simulink model "spwm_3_class3"  (R2024b)
settings: Solver=VariableStepAuto  StartTime=0.0  StopTime=1/50  RelTol=1e-3
libraries: spsTriangleGeneratorLib x1
settings Model: Creator=vasudha  LastModifiedBy=vasudha

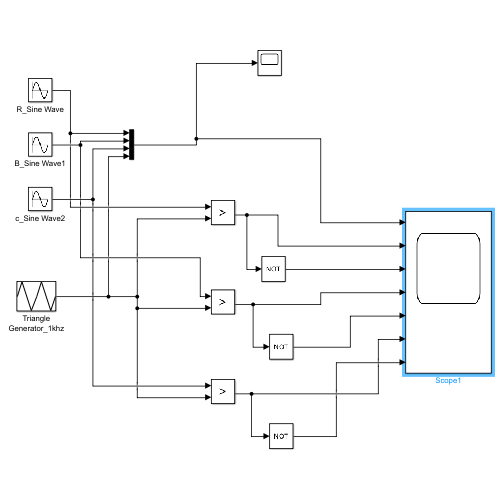
[thumbnail: Simulink's stored preview of the top-level diagram]
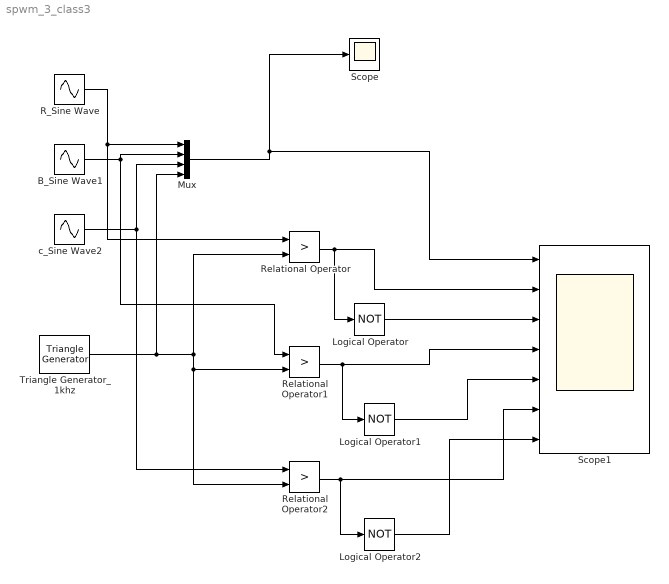
== system spwm_3_class3 ==
  B_Sine Wave1 : Sin  Amplitude=0.8  Frequency=314  Phase=2.10  SampleTime=0
  Logical Operator : Logic  Operator=NOT  AllPortsSameDT=off  OutDataTypeStr=boolean
  Logical Operator1 : Logic  Operator=NOT  AllPortsSameDT=off  OutDataTypeStr=boolean
  Logical Operator2 : Logic  Operator=NOT  AllPortsSameDT=off  OutDataTypeStr=boolean
  Mux : Mux
  R_Sine Wave : Sin  Amplitude=0.8  Frequency=314  SampleTime=0
  Relational Operator : RelationalOperator  Operator=>  OutDataTypeStr=boolean  RndMeth=Simplest  InputSameDT=off
  Relational Operator1 : RelationalOperator  Operator=>  OutDataTypeStr=boolean  RndMeth=Simplest  InputSameDT=off
  Relational Operator2 : RelationalOperator  Operator=>  OutDataTypeStr=boolean  RndMeth=Simplest  InputSameDT=off
  Scope : Scope
  Scope1 : Scope  NumInputPorts=7
  Triangle Generator_1khz : spsTriangleGeneratorLib/Triangle Generator  Freq=1e3  Phase=90  Ts=0
  c_Sine Wave2 : Sin  Amplitude=0.8  Frequency=314  Phase=-2.10  SampleTime=0
  wires:
  R_Sine Wave/1 -> Relational Operator/1, Mux/1
  B_Sine Wave1/1 -> Relational Operator1/1, Mux/2
  c_Sine Wave2/1 -> Relational Operator2/1, Mux/3
  Mux/1 -> Scope/1, Scope1/1
  Triangle Generator_1khz/1 -> Mux/4, Relational Operator2/2, Relational Operator1/2, Relational Operator/2
  Relational Operator/1 -> Logical Operator/1, Scope1/2
  Logical Operator/1 -> Scope1/3
  Relational Operator1/1 -> Logical Operator1/1, Scope1/4
  Logical Operator1/1 -> Scope1/5
  Relational Operator2/1 -> Logical Operator2/1, Scope1/6
  Logical Operator2/1 -> Scope1/7
